simulink model "TP3DC"  (R2019a)
settings: Solver=VariableStepAuto  StartTime=0.0  StopTime=10.0  RelTol=1e-3
values from neighbouring files (symbols this model uses):
  A = [1 dt;0 1]    [TP3Combined_Main.m]    (also in TP3DC_Main.m; TP3Q3_Main.m)
  B = [dt*dt/2;dt]    [TP3Combined_Main.m]    (also in TP3DC_Main.m; TP3Q3_Main.m)
  dt = 0.001    [TP3Au422_Main.m]    (also in TP3Combined_Main.m; TP3DC_Main.m; TP3Q3_Main.m)
  F_dis1 = 150    [TP3Au422_Main.m]    (also in TP3Combined_Main.m; TP3DC_Main.m; TP3Q3_Main.m)
  F_dis2 = -107.5    [TP3Au422_Main.m]    (also in TP3Combined_Main.m; TP3DC_Main.m; TP3Q3_Main.m)
  H = [1 0;0 1]    [TP3Combined_Main.m]    (also in TP3DC_Main.m; TP3Q3_Main.m)
  Kd = 5    [TP3Au422_Main.m]    (also in TP3Combined_Main.m = 3; TP3DC_Main.m = 3; TP3Q3_Main.m = 3)
  Kp = 50    [TP3Au422_Main.m]    (also in TP3Combined_Main.m = 6; TP3DC_Main.m = 6; TP3Q3_Main.m = 6)
  m = 1    [TP3Au422_Main.m]    (also in TP3Combined_Main.m; TP3DC_Main.m; TP3Q3_Main.m)
  P0 = [VarianceU^2 0;0 VarianceA^2]    [TP3Combined_Main.m]    (also in TP3DC_Main.m; TP3Q3_Main.m)
  Q = [0.0001 0;0 2]    [TP3Combined_Main.m]    (also in TP3DC_Main.m; TP3Q3_Main.m)
  R = [VarianceU^2 0;0 0.075]    [TP3Combined_Main.m]    (also in TP3DC_Main.m; TP3Q3_Main.m)
  t_dis1 = 20    [TP3Au422_Main.m]    (also in TP3Combined_Main.m; TP3DC_Main.m; TP3Q3_Main.m)
  t_dis2 = 40    [TP3Au422_Main.m]    (also in TP3Combined_Main.m; TP3DC_Main.m; TP3Q3_Main.m)
  VarianceA = 0.075    [TP3Combined_Main.m]    (also in TP3DC_Main.m; TP3Q3_Main.m)
  VarianceU = 0.0000075    (= 7.5e-06)    [TP3Combined_Main.m]    (also in TP3DC_Main.m; TP3Q3_Main.m)
  xp0 = 0    [TP3Combined_Main.m]    (also in TP3DC_Main.m; TP3Q3_Main.m)
  xv0 = 0    [TP3Combined_Main.m]    (also in TP3DC_Main.m; TP3Q3_Main.m)
  zd = 2    [TP3Au422_Main.m]    (also in TP3Combined_Main.m; TP3DC_Main.m; TP3Q3_Main.m)
libraries: dspsrcs4 x3
settings Model: Creator=Huynh  LastModifiedBy=Huynh

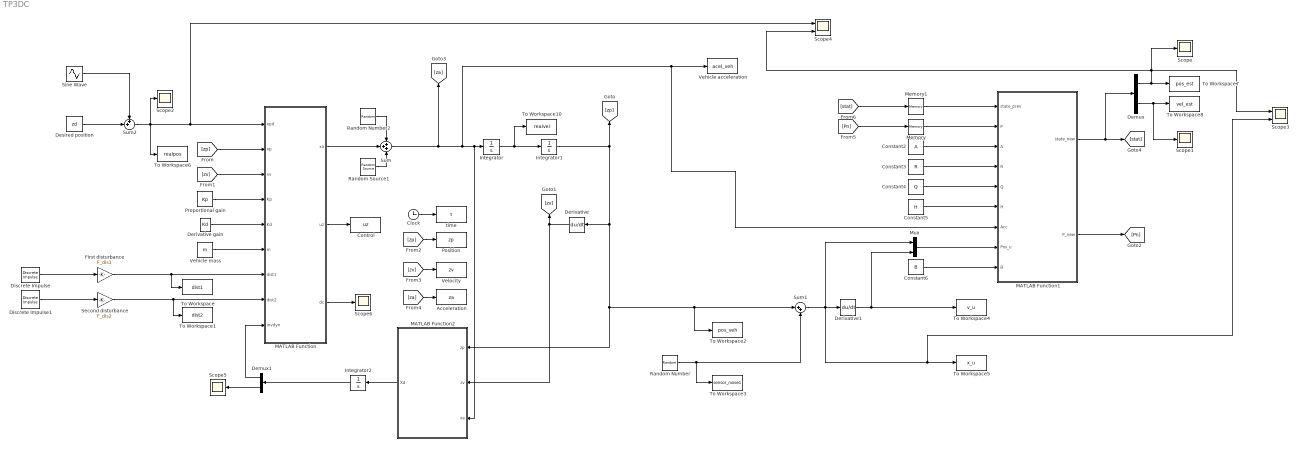
== system TP3DC ==
  Acceleration : ToWorkspace  VariableName=za  SampleTime=dt
  Clock : Clock
  Constant2 : Constant  Value=A
  Constant3 : Constant  Value=R
  Constant4 : Constant  Value=Q
  Constant5 : Constant  Value=H
  Constant6 : Constant  Value=B
  Control : ToWorkspace  VariableName=uz  SampleTime=dt
  Demux : Demux  Outputs=2
  Demux1 : Demux  Outputs=2
  Derivative : Derivative
  Derivative gain : Constant  Value=Kd
  Derivative1 : Derivative
  Desired position : Constant  Value=zd
  Discrete Impulse : dspsrcs4/Discrete  Impulse  Delay=t_dis1/dt  SampleTime=dt  FrameSample=1  OutputFrames=off  dataType=double  isSigned=on  wordLen=16  udDataType=sfix(16)  fracBitsMode=Best precision  numFracBits=15  OutDataTypeStr=double  LastOutDataTypeStr=double
  Discrete Impulse1 : dspsrcs4/Discrete  Impulse  Delay=t_dis2/dt  SampleTime=dt  FrameSample=1  OutputFrames=off  dataType=double  isSigned=on  wordLen=16  udDataType=sfix(16)  fracBitsMode=Best precision  numFracBits=15  OutDataTypeStr=double  LastOutDataTypeStr=double
  First disturbance : Gain  Gain=F_dis1
  Integrator : Integrator
  Integrator1 : Integrator
  Integrator2 : Integrator  InitialCondition=[0 0]
  MATLAB Function : MATLAB Function  TreatAsAtomicUnit=on
  MATLAB Function1 : MATLAB Function  TreatAsAtomicUnit=on
  MATLAB Function2 : MATLAB Function  TreatAsAtomicUnit=on
  Memory : Memory  InitialCondition=P0
  Memory1 : Memory  InitialCondition=[xp0;xv0]
  Mux : Mux  Inputs=2
  Position : ToWorkspace  VariableName=zp  SampleTime=dt
  Proportional gain : Constant  Value=Kp
  Random Number : RandomNumber  Variance=VarianceU  SampleTime=dt
  Random Number2 : RandomNumber  Variance=VarianceA  SampleTime=dt
  Random Source1 : dspsrcs4/Random Source  SrcType=Uniform  NormMethod=Ziggurat  CltLength=12  MinVal=Min  MaxVal=Max  MeanVal=0  VarVal=1  RepMode=Not repeatable  rawSeed=1  IsInherit=off  SampMode=Discrete  SampTime=Bias_Sample_time  SampFrame=1  DataType=Double  OutComplex=Real  OutputFrames=off
  Scope{,1..2,5..6} (5 alike) : Scope
  Scope3 : Scope  NumInputPorts=2
  Scope4 : Scope  NumInputPorts=2
  Second disturbance : Gain  Gain=F_dis2
  Sine Wave : Sin  Frequency=2/3/t_sim  SampleTime=dt
  Sum : Sum  Inputs=+++
  Sum1 : Sum  Inputs=|++
  Sum2 : Sum  Inputs=++|
  To Workspace : ToWorkspace  VariableName=dist1  SampleTime=dt
      settings: Save2DSignal=2-D array (concatenate along first dimension)
  To Workspace1 : ToWorkspace  VariableName=dist2  SampleTime=dt
      settings: Save2DSignal=2-D array (concatenate along first dimension)
  To Workspace10 : ToWorkspace  VariableName=realvel  SampleTime=dt
      settings: Save2DSignal=2-D array (concatenate along first dimension)
  To Workspace2 : ToWorkspace  VariableName=pos_veh  SampleTime=dt
      settings: Save2DSignal=2-D array (concatenate along first dimension)
  To Workspace3 : ToWorkspace  VariableName=sensor_noise1  SampleTime=dt
      settings: Save2DSignal=2-D array (concatenate along first dimension)
  To Workspace4 : ToWorkspace  VariableName=v_u  SampleTime=dt
      settings: Save2DSignal=2-D array (concatenate along first dimension)
  To Workspace5 : ToWorkspace  VariableName=x_u  SampleTime=dt
      settings: Save2DSignal=2-D array (concatenate along first dimension)
  To Workspace6 : ToWorkspace  VariableName=realpos  SampleTime=dt
      settings: Save2DSignal=2-D array (concatenate along first dimension)
  To Workspace7 : ToWorkspace  VariableName=pos_est  SampleTime=dt
      settings: Save2DSignal=2-D array (concatenate along first dimension)
  To Workspace8 : ToWorkspace  VariableName=vel_est  SampleTime=dt
      settings: Save2DSignal=2-D array (concatenate along first dimension)
  "Vehicle acceleration " : ToWorkspace  VariableName=acel_veh  SampleTime=dt
      settings: Save2DSignal=2-D array (concatenate along first dimension)
  Vehicle mass : Constant  Value=m
  Velocity : ToWorkspace  VariableName=zv  SampleTime=dt
  time : ToWorkspace  VariableName=t  SampleTime=dt
  wires:
  [za] -> Acceleration/1
  Sum2/1 -> To Workspace6/1, Scope2/1, Scope4/1, MATLAB Function/1(xpd)
  MATLAB Function/1(xa) -> Sum/2
  Sine Wave/1 -> Sum2/1
  Desired position/1 -> Sum2/2
  Mux/1 -> MATLAB Function1/8(Pos_u)
  Discrete Impulse1/1 -> Second disturbance/1
  First disturbance/1 -> To Workspace/1, MATLAB Function/7(dist1)
  Sum/1 -> MATLAB Function2/3(xa), Integrator/1, MATLAB Function1/7(Acc), "Vehicle acceleration "/1, [za]
  Discrete Impulse/1 -> First disturbance/1
  Random Number2/1 -> Sum/1
  Demux/2 -> Scope1/1, To Workspace8/1
  Clock/1 -> time/1
  [zv] -> Velocity/1
  Memory/1 -> MATLAB Function1/2(P)
  Constant2/1 -> MATLAB Function1/3(A)
  Constant5/1 -> MATLAB Function1/6(H)
  Derivative gain/1 -> MATLAB Function/5(Kd)
  Integrator/1 -> To Workspace10/1, Integrator1/1
  Derivative/1 -> [zv], MATLAB Function2/2(zv)
  Second disturbance/1 -> To Workspace1/1, MATLAB Function/8(dist2)
  Derivative1/1 -> Mux/2, To Workspace4/1
  [zv] -> MATLAB Function/3(xv)
  Constant4/1 -> MATLAB Function1/5(Q)
  Sum1/1 -> Mux/1, Scope3/2, To Workspace5/1, Derivative1/1
  Constant3/1 -> MATLAB Function1/4(R)
  Memory1/1 -> MATLAB Function1/1(state_prev)
  [Pn] -> Memory/1
  [zp] -> Position/1
  [stat] -> Memory1/1
  Vehicle mass/1 -> MATLAB Function/6(m)
  [zp] -> MATLAB Function/2(xp)
  MATLAB Function/2(uz) -> Control/1
  Random Number/1 -> To Workspace3/1, Sum1/2
  Constant6/1 -> MATLAB Function1/9(B)
  Integrator1/1 -> MATLAB Function2/1(zp), Sum1/1, To Workspace2/1, Derivative/1, [zp]
  MATLAB Function1/2(P_new) -> [Pn]
  Proportional gain/1 -> MATLAB Function/4(Kp)
  Random Source1/1 -> Sum/3
  Demux/1 -> Scope4/2, Scope3/1, Scope/1, To Workspace7/1
  MATLAB Function1/1(state_new) -> Demux/1, [stat]
  MATLAB Function2/1(Xd) -> Integrator2/1
  Integrator2/1 -> Demux1/1
  Demux1/2 -> Scope5/1
  Demux1/1 -> MATLAB Function/9(invdyn)
  MATLAB Function/3(dc) -> Scope6/1

== matlab function TP3DC/MATLAB Function1 ==
  data: state_prev input; state_new output; P input; A input; R input; Q input; H input; Acc input; Pos_u input; B input; P_new output
function [state_new, P_new] = KalmanFilterWithBias(state_prev, P, A, R, Q, H, Acc, Pos_u, B) 
%% Estimation of prediction phase
state_est = A*state_prev+B*Acc;
P_est = A*P*A'+Q;
K=P_est*H'*inv(H*P_est*H'+R);

%% Correction phase
Measu=Pos_u;
state=state_est+K*(Measu-H*state_est);
P_new=(1-K*H)*P_est;

%%
state_new = state;

== matlab function TP3DC/MATLAB Function ==
  data: xpd input; xa output; xp input; xv input; Kp input; Kd input; m input; dist1 input; dist2 input; uz output; invdyn input; dc output
function [xa, uz, dc] = PD(xpd, xp, xv, Kp, Kd, m, dist1, dist2, invdyn) %PD Function

exp = xpd - xp; %Position error
exv = 0 - xv; %Velocity error
dc = 1.1*invdyn - xp;
uz = Kp * (exp + dc) + Kd * exv + 9.81 * m; %Control law equation
if uz > 20
    uz = 20;
elseif uz < -10
    uz = -10;
end
xa = (uz + dist1 + dist2 - 9.81 * m) / m ; %Acceleration update with disturbances

== matlab function TP3DC/MATLAB Function2 ==
  data: zp input; Xd output; zv input; xa input
function Xd = InvDyn(zp, zv, xa)
X = [zp, zv];
Xd = [zv, xa];
